simulink model "LoopCounter"  (R2022b)
settings: Solver=VariableStepAuto  StartTime=0.0  StopTime=10.0  RelTol=1e-3
settings Model: Creator=iceki  LastModifiedBy=iceki

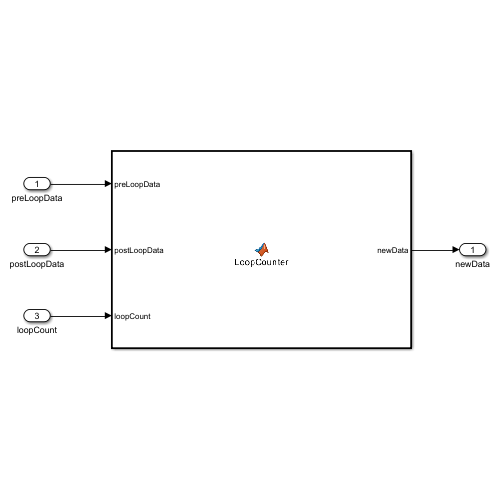
[thumbnail: Simulink's stored preview of the top-level diagram]
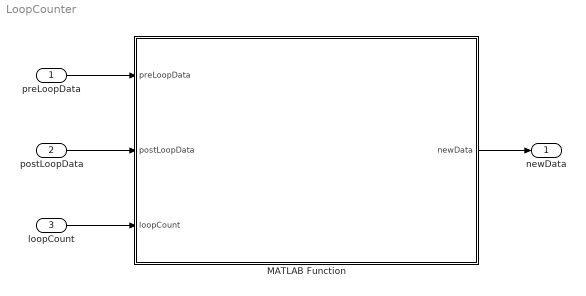
== system LoopCounter ==
  preLoopData : Inport
  postLoopData : Inport  Port=2
  loopCount : Inport  Port=3
  MATLAB Function : MATLAB Function  TreatAsAtomicUnit=on
  newData : Outport
  wires:
  preLoopData/1 -> MATLAB Function/1(preLoopData)
  postLoopData/1 -> MATLAB Function/2(postLoopData)
  MATLAB Function/1(newData) -> newData/1
  loopCount/1 -> MATLAB Function/3(loopCount)

== matlab function LoopCounter/MATLAB Function ==
  data: preLoopData input; newData output; postLoopData input; loopCount input
function newData = LoopCounter(preLoopData,postLoopData,loopCount)
% Function to count time generated by loops, assuming each module
% time has been estimated already.
%
% Written by: Darian Muresan
% Modified last: October 12, 2023
newData = preLoopData+loopCount*(postLoopData-preLoopData);
